simulink library "working_reference_library"  (Simulink 7.9)
settings: Solver=ode45  StartTime=0.0  StopTime=10.0  RelTol=1e-3
undefined symbols (not defined in the file or in its folder): fbaud, fphasej, fsscj, PhaseJ, SSCJ
libraries: simulink_extras x40, working_reference_library x12
Description:
  | Working reference library
settings Model: Creator=asus  LastModifiedBy=asus

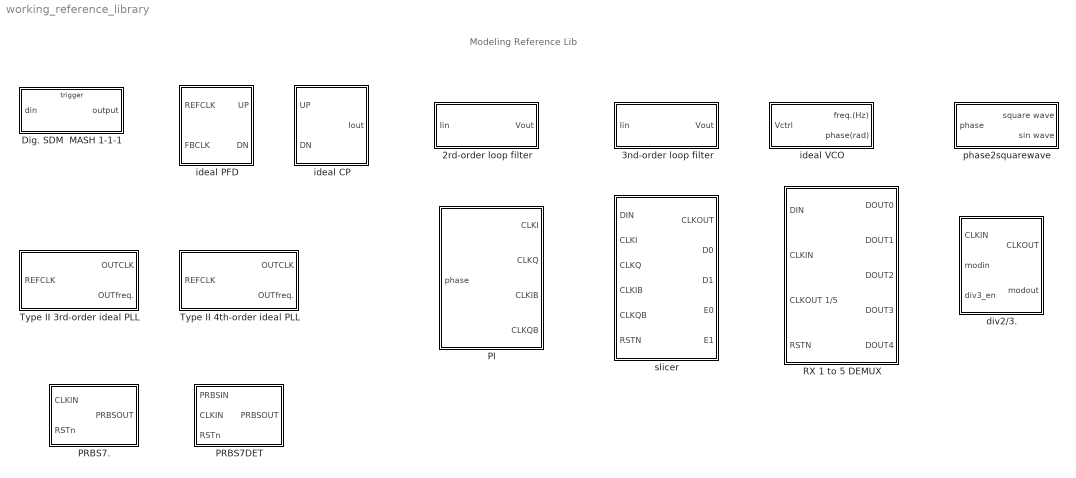
== system working_reference_library ==
  note: Modeling Reference Lib
  2rd-order loop filter : Subsystem  mask{R1=7.5e3, C1=180e-12, C2=4e-12}
      mask prompts: R1 "zero resistor R1(ohm)"; C1 "zero capacitance C1(F)"; C2 "pole capacitance C2(F)"
  3nd-order loop filter : Subsystem  mask{R1=6e3, C1=150e-12, C2=3e-12, R3=6e3*2, C3=1e-12}
      mask prompts: R1 "zero resistor R1(ohm)"; C1 "zero capacitance C1(F)"; C2 "pole1 capacitance C2(F)"; R3 "pole2 resistor R3(ohm)"; C3 "pole2 capacitance C3(F)"
  Dig. SDM  MASH 1-1-1 : Subsystem  TreatAsAtomicUnit=on  mask{N=9}
      mask prompts: N "bit-width for input"
  PI : Subsystem
  PRBS7. : Subsystem
  PRBS7DET : Subsystem
  RX 1 to 5 DEMUX : Subsystem
  Type II 3rd-order ideal PLL : Subsystem  mask{delay=100e-12, Icp=20e-6, R1=6e3, C1=180e-12, C2=4e-12, f_free=1.4e9, Kvco=700e6, Ndiv=15}
      mask prompts: delay "PFD Reset Delay--delay(s)"; Icp "Charge Pump Current--Icp(A)"; R1 "Loop Filter Zero Resistor--R1(ohm)"; C1 "Loop Filter Zero Capacitance--C1(F)"; C2 "Loop Filter Pole Capacitance--C2(F)"; f_free "VCO free running freqency--f_free(Hz)"; Kvco "VCO gain--Kvco(Hz/V)"; Ndiv "Divider Mod--Ndiv"
  Type II 4th-order ideal PLL : Subsystem  mask{delay=100e-12, Icp=20e-6, R1=6e3, C1=180e-12, C2=4e-12, R3=12e3, C3=2e-12, f_free=1.4e9, Kvco=700e6, Ndiv=15}
      mask prompts: delay "PFD Reset Delay--delay(s)"; Icp "Charge Pump Current--Icp(A)"; R1 "Loop Filter Zero resistor--R1(ohm)"; C1 "Loop Filter Zero Capacitance--C1(F)"; C2 "Loop Filter 1st-pole Capacitance--C2(F)"; R3 "Loop Filter 2nd-pole Resistor--R3(ohm)"; C3 "Loop Filter 2nd-pole Capacitance--C3(F)"; f_free "VCO free running freqency--f_free(Hz)"; Kvco "VCO gain--Kvco(Hz/V)"; Ndiv "Divider Mod--Ndiv"
  div2/3. : Subsystem
  ideal CP : Subsystem  mask{Icp=20e-6}
      mask prompts: Icp "charge pump current(A)"
  ideal PFD : Subsystem  mask{delay=100e-12}
      mask prompts: delay "reset delay"
  ideal VCO : Subsystem  mask{f_free=1.4e9, Kvco=700e6}
      mask prompts: f_free "free running freq.(Hz)"; Kvco "VCO gain(Hz/V)"
  phase2squarewave : Subsystem
  slicer : Subsystem  TreatAsAtomicUnit=on

== system working_reference_library/2rd-order loop filter ==
  Iin : Inport
  Data Type Conversion : DataTypeConversion  OutDataTypeStr=double
  Transfer Fcn : TransferFcn  Numerator=[R1*C1 1]  Denominator=[C2*R1*C1 (C1+C2) 0]  AbsoluteTolerance=1e-12
  Vout : Outport
  wires:
  Data Type Conversion/1 -> Transfer Fcn/1
  Transfer Fcn/1 -> Vout/1
  Iin/1 -> Data Type Conversion/1

== system working_reference_library/3nd-order loop filter ==
  Iin : Inport
  Data Type Conversion : DataTypeConversion  OutDataTypeStr=double
  Transfer Fcn : TransferFcn  Numerator=[R1*C1 1]  Denominator=[C2*R1*C1*R3*C3 (C1*R3*C3+C3*R1*C1+C2*(R1*C1+R3*C3)) (C1+C2+C3) 0]  AbsoluteTolerance=1e-12
  Vout : Outport
  wires:
  Iin/1 -> Data Type Conversion/1
  Transfer Fcn/1 -> Vout/1
  Data Type Conversion/1 -> Transfer Fcn/1

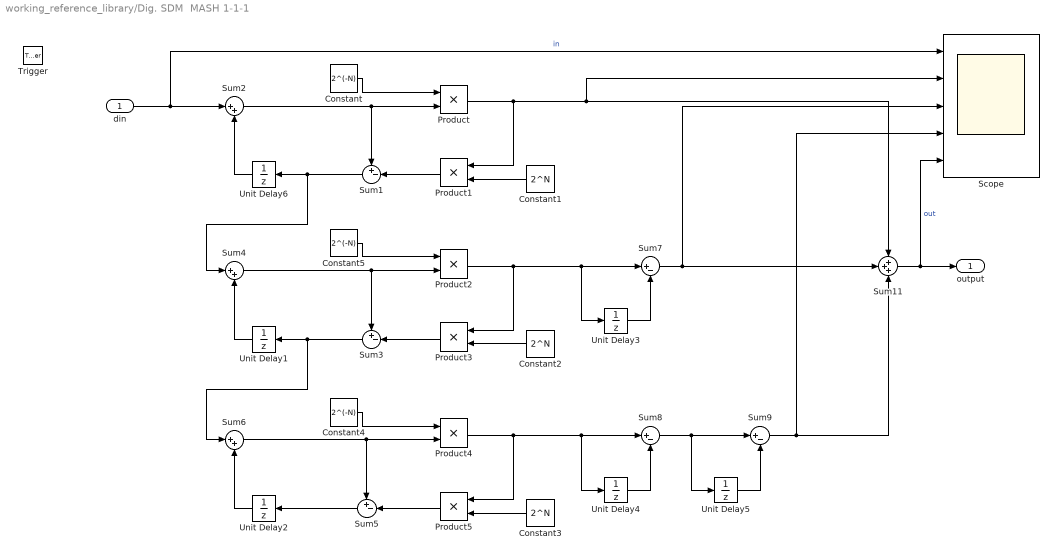
== system working_reference_library/Dig. SDM  MASH 1-1-1 ==
  din : Inport
  Trigger : TriggerPort
  Constant : Constant  Value=2^(-N)
  Constant1 : Constant  Value=2^N
  Constant2 : Constant  Value=2^N
  Constant3 : Constant  Value=2^N
  Constant4 : Constant  Value=2^(-N)
  Constant5 : Constant  Value=2^(-N)
  Product : Product  OutDataTypeStr=int8  RndMeth=Zero
  Product1 : Product  RndMeth=Zero
  Product2 : Product  OutDataTypeStr=int8  RndMeth=Zero
  Product3 : Product  RndMeth=Zero
  Product4 : Product  OutDataTypeStr=int8  RndMeth=Zero
  Product5 : Product  RndMeth=Zero
  Scope : Scope  NumInputPorts=5
      settings: YMin=-100~0~-5~-5~-5  YMax=600~1~5~5~5  MaxDataPoints=500000
  Sum1 : Sum  Inputs=+-|
  Sum11 : Sum  Inputs=+++
  Sum2 : Sum  Inputs=|++
  Sum3 : Sum  Inputs=+-|
  Sum4 : Sum  Inputs=|++
  Sum5 : Sum  Inputs=+-|
  Sum6 : Sum  Inputs=|++
  Sum7 : Sum  Inputs=|+-
  Sum8 : Sum  Inputs=|+-
  Sum9 : Sum  Inputs=|+-
  Unit Delay{1..6} (6 alike) : UnitDelay  SampleTime=-1
  output : Outport
  wires:
  Constant/1 -> Product/1
  Product/1 -> Product1/1, Sum11/1, Scope/2
  Constant1/1 -> Product1/2
  Product1/1 -> Sum1/2
  din/1 -> Sum2/1, Scope/1  "in"
  Sum11/1 -> output/1, Scope/5  "out"
  Unit Delay6/1 -> Sum2/2
  Sum2/1 -> Sum1/1, Product/2
  Constant5/1 -> Product2/1
  Product2/1 -> Product3/1, Sum7/1, Unit Delay3/1
  Constant2/1 -> Product3/2
  Product3/1 -> Sum3/2
  Unit Delay1/1 -> Sum4/2
  Sum4/1 -> Sum3/1, Product2/2
  Constant4/1 -> Product4/1
  Product4/1 -> Product5/1, Sum8/1, Unit Delay4/1
  Constant3/1 -> Product5/2
  Unit Delay2/1 -> Sum6/2
  Sum6/1 -> Sum5/1, Product4/2
  Unit Delay3/1 -> Sum7/2
  Unit Delay4/1 -> Sum8/2
  Sum8/1 -> Sum9/1, Unit Delay5/1
  Unit Delay5/1 -> Sum9/2
  Sum9/1 -> Sum11/3, Scope/4
  Sum7/1 -> Sum11/2, Scope/3
  Sum1/1 -> Unit Delay6/1, Sum4/1
  Product5/1 -> Sum5/2
  Sum5/1 -> Unit Delay2/1
  Sum3/1 -> Unit Delay1/1, Sum6/1

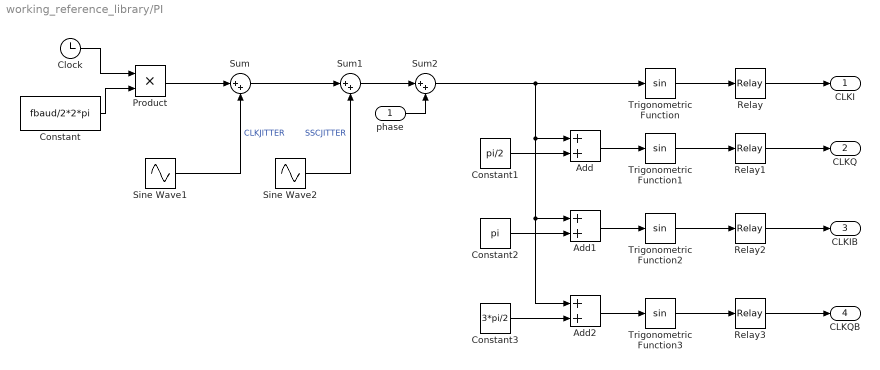
== system working_reference_library/PI ==
  phase : Inport
  Add : Sum
  Add1 : Sum
  Add2 : Sum
  Clock : Clock
  Constant : Constant  Value=fbaud/2*2*pi
  Constant1 : Constant  Value=pi/2
  Constant2 : Constant  Value=pi
  Constant3 : Constant  Value=3*pi/2
  Product : Product  RndMeth=Zero
  Relay{,1..3} (4 alike) : Relay  OnSwitchValue=0.5  OffSwitchValue=-0.5
  Sine Wave1 : Sin  Amplitude=PhaseJ  Frequency=fphasej*2*pi  SampleTime=0
  Sine Wave2 : Sin  Amplitude=SSCJ  Frequency=fsscj*2*pi  SampleTime=0
  Sum : Sum  Inputs=|++
  Sum1 : Sum  Inputs=|++
  Sum2 : Sum  Inputs=|++
  Trigonometric Function{,1..3} (4 alike) : Trigonometry
  CLKI : Outport
  CLKQ : Outport  Port=2
  CLKIB : Outport  Port=3
  CLKQB : Outport  Port=4
  wires:
  Sum2/1 -> Add2/1, Add1/1, Add/1, Trigonometric Function/1
  phase/1 -> Sum2/2
  Sum1/1 -> Sum2/1
  Relay3/1 -> CLKQB/1
  Relay2/1 -> CLKIB/1
  Relay1/1 -> CLKQ/1
  Relay/1 -> CLKI/1
  Add2/1 -> Trigonometric Function3/1
  Trigonometric Function3/1 -> Relay3/1
  Constant3/1 -> Add2/2
  Add1/1 -> Trigonometric Function2/1
  Trigonometric Function2/1 -> Relay2/1
  Constant2/1 -> Add1/2
  Add/1 -> Trigonometric Function1/1
  Trigonometric Function1/1 -> Relay1/1
  Constant1/1 -> Add/2
  Trigonometric Function/1 -> Relay/1
  Sine Wave2/1 -> Sum1/2  "SSCJITTER"
  Sum/1 -> Sum1/1
  Sine Wave1/1 -> Sum/2  "CLKJITTER"
  Product/1 -> Sum/1
  Constant/1 -> Product/2
  Clock/1 -> Product/1

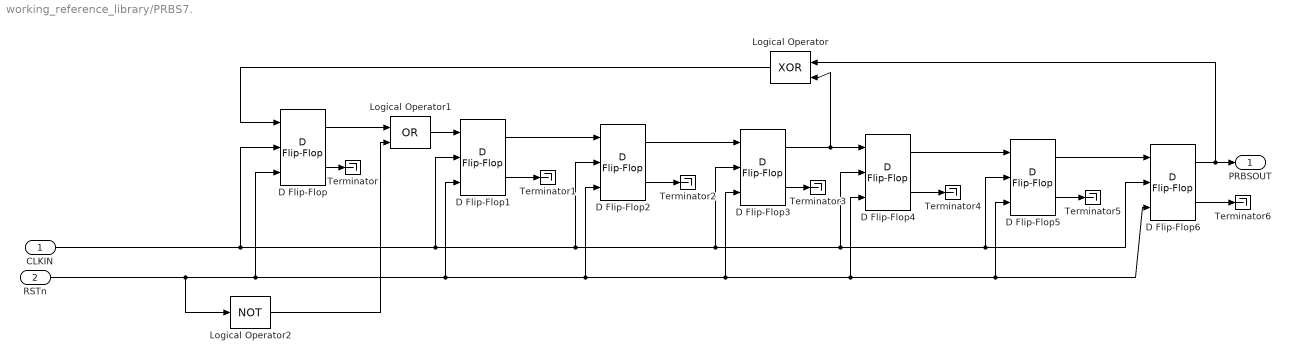
== system working_reference_library/PRBS7. ==
  CLKIN : Inport
  RSTn : Inport  Port=2
  D Flip-Flop{,1..6} (7 alike) : simulink_extras/Flip Flops/D Flip-Flop
  Logical Operator : Logic  Operator=XOR  IconShape=distinctive  AllPortsSameDT=off  OutDataTypeStr=boolean
  Logical Operator1 : Logic  Operator=OR  IconShape=distinctive  AllPortsSameDT=off  OutDataTypeStr=boolean
  Logical Operator2 : Logic  Operator=NOT  IconShape=distinctive  AllPortsSameDT=off  OutDataTypeStr=boolean
  Terminator{,1..6} (7 alike) : Terminator
  PRBSOUT : Outport
  wires:
  Logical Operator2/1 -> Logical Operator1/2
  D Flip-Flop/1 -> Logical Operator1/1
  Logical Operator1/1 -> D Flip-Flop1/1
  D Flip-Flop6/1 -> Logical Operator/1, PRBSOUT/1
  D Flip-Flop6/2 -> Terminator6/1
  D Flip-Flop5/2 -> Terminator5/1
  D Flip-Flop4/2 -> Terminator4/1
  D Flip-Flop3/2 -> Terminator3/1
  D Flip-Flop5/1 -> D Flip-Flop6/1
  D Flip-Flop4/1 -> D Flip-Flop5/1
  D Flip-Flop3/1 -> D Flip-Flop4/1, Logical Operator/2
  RSTn/1 -> D Flip-Flop6/3, D Flip-Flop5/3, D Flip-Flop4/3, D Flip-Flop3/3, D Flip-Flop2/3, D Flip-Flop1/3, D Flip-Flop/3, Logical Operator2/1
  D Flip-Flop2/2 -> Terminator2/1
  D Flip-Flop2/1 -> D Flip-Flop3/1
  D Flip-Flop1/2 -> Terminator1/1
  D Flip-Flop1/1 -> D Flip-Flop2/1
  D Flip-Flop/2 -> Terminator/1
  CLKIN/1 -> D Flip-Flop/2, D Flip-Flop1/2, D Flip-Flop2/2, D Flip-Flop3/2, D Flip-Flop4/2, D Flip-Flop6/2, D Flip-Flop5/2
  Logical Operator/1 -> D Flip-Flop/1

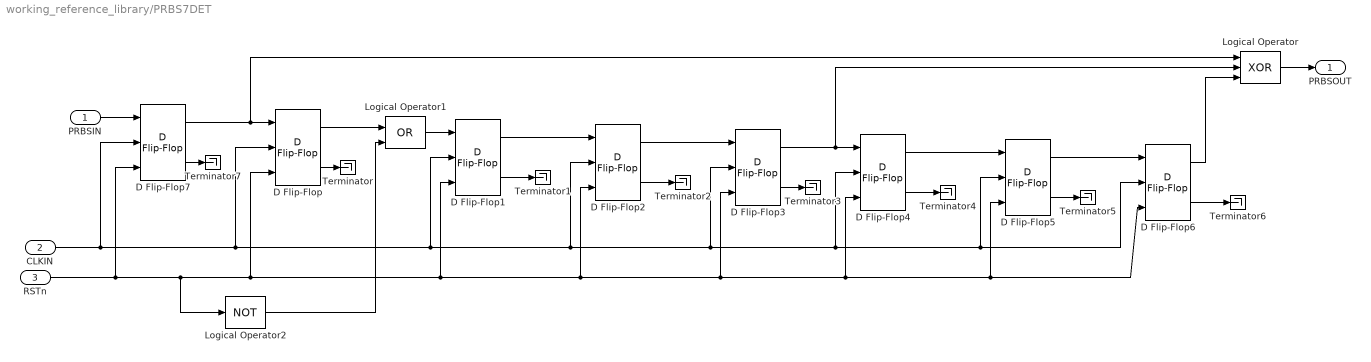
== system working_reference_library/PRBS7DET ==
  PRBSIN : Inport
  CLKIN : Inport  Port=2
  RSTn : Inport  Port=3
  D Flip-Flop{,1..7} (8 alike) : simulink_extras/Flip Flops/D Flip-Flop
  Logical Operator : Logic  Operator=XOR  Inputs=3  IconShape=distinctive  AllPortsSameDT=off  OutDataTypeStr=boolean
  Logical Operator1 : Logic  Operator=OR  IconShape=distinctive  AllPortsSameDT=off  OutDataTypeStr=boolean
  Logical Operator2 : Logic  Operator=NOT  IconShape=distinctive  AllPortsSameDT=off  OutDataTypeStr=boolean
  Terminator{,1..7} (8 alike) : Terminator
  PRBSOUT : Outport
  wires:
  CLKIN/1 -> D Flip-Flop5/2, D Flip-Flop6/2, D Flip-Flop4/2, D Flip-Flop3/2, D Flip-Flop2/2, D Flip-Flop1/2, D Flip-Flop/2, D Flip-Flop7/2
  D Flip-Flop/2 -> Terminator/1
  D Flip-Flop1/1 -> D Flip-Flop2/1
  D Flip-Flop1/2 -> Terminator1/1
  D Flip-Flop2/1 -> D Flip-Flop3/1
  D Flip-Flop2/2 -> Terminator2/1
  RSTn/1 -> Logical Operator2/1, D Flip-Flop/3, D Flip-Flop1/3, D Flip-Flop2/3, D Flip-Flop3/3, D Flip-Flop4/3, D Flip-Flop5/3, D Flip-Flop6/3, D Flip-Flop7/3
  D Flip-Flop3/1 -> D Flip-Flop4/1, Logical Operator/2
  D Flip-Flop4/1 -> D Flip-Flop5/1
  D Flip-Flop5/1 -> D Flip-Flop6/1
  D Flip-Flop3/2 -> Terminator3/1
  D Flip-Flop4/2 -> Terminator4/1
  D Flip-Flop5/2 -> Terminator5/1
  D Flip-Flop6/2 -> Terminator6/1
  D Flip-Flop6/1 -> Logical Operator/3
  Logical Operator1/1 -> D Flip-Flop1/1
  D Flip-Flop/1 -> Logical Operator1/1
  Logical Operator2/1 -> Logical Operator1/2
  D Flip-Flop7/1 -> D Flip-Flop/1, Logical Operator/1
  D Flip-Flop7/2 -> Terminator7/1
  Logical Operator/1 -> PRBSOUT/1
  PRBSIN/1 -> D Flip-Flop7/1

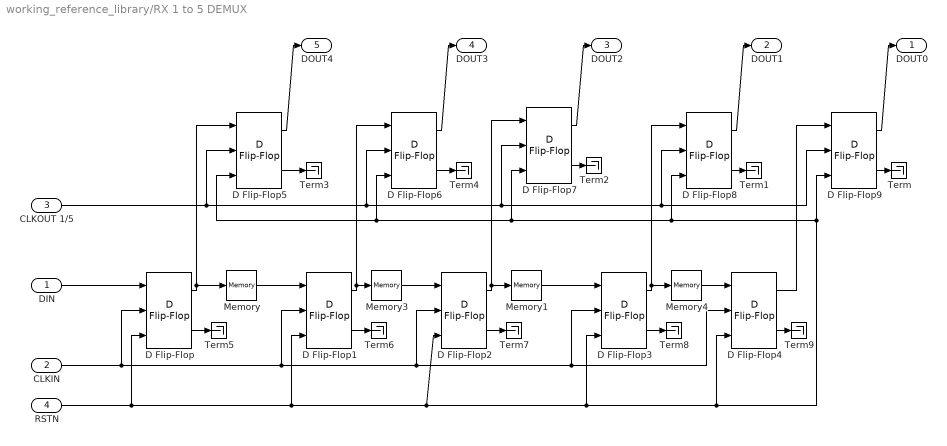
== system working_reference_library/RX 1 to 5 DEMUX ==
  DIN : Inport
  CLKIN : Inport  Port=2
  CLKOUT 1/5 : Inport  Port=3
  RSTN : Inport  Port=4
  D Flip-Flop{,1..9} (10 alike) : simulink_extras/Flip Flops/D Flip-Flop
  Memory{,1,3..4} (4 alike) : Memory
  Term{,1..9} (10 alike) : Terminator
  DOUT0 : Outport
  DOUT1 : Outport  Port=2
  DOUT2 : Outport  Port=3
  DOUT3 : Outport  Port=4
  DOUT4 : Outport  Port=5
  wires:
  DIN/1 -> D Flip-Flop/1
  D Flip-Flop/1 -> Memory/1, D Flip-Flop5/1
  Memory/1 -> D Flip-Flop1/1
  D Flip-Flop1/1 -> D Flip-Flop6/1, Memory3/1
  D Flip-Flop2/1 -> D Flip-Flop7/1, Memory1/1
  Memory1/1 -> D Flip-Flop3/1
  D Flip-Flop3/1 -> D Flip-Flop8/1, Memory4/1
  Memory3/1 -> D Flip-Flop2/1
  Memory4/1 -> D Flip-Flop4/1
  D Flip-Flop5/1 -> DOUT4/1
  D Flip-Flop4/1 -> D Flip-Flop9/1
  D Flip-Flop6/1 -> DOUT3/1
  D Flip-Flop7/1 -> DOUT2/1
  D Flip-Flop8/1 -> DOUT1/1
  D Flip-Flop9/1 -> DOUT0/1
  CLKOUT 1/5/1 -> D Flip-Flop9/2, D Flip-Flop8/2, D Flip-Flop7/2, D Flip-Flop6/2, D Flip-Flop5/2
  CLKIN/1 -> D Flip-Flop4/2, D Flip-Flop3/2, D Flip-Flop2/2, D Flip-Flop1/2, D Flip-Flop/2
  RSTN/1 -> D Flip-Flop/3, D Flip-Flop1/3, D Flip-Flop2/3, D Flip-Flop3/3, D Flip-Flop4/3, D Flip-Flop9/3, D Flip-Flop8/3, D Flip-Flop7/3, D Flip-Flop5/3, D Flip-Flop6/3
  D Flip-Flop9/2 -> Term/1
  D Flip-Flop7/2 -> Term2/1
  D Flip-Flop5/2 -> Term3/1
  D Flip-Flop6/2 -> Term4/1
  D Flip-Flop8/2 -> Term1/1
  D Flip-Flop4/2 -> Term9/1
  D Flip-Flop3/2 -> Term8/1
  D Flip-Flop2/2 -> Term7/1
  D Flip-Flop1/2 -> Term6/1
  D Flip-Flop/2 -> Term5/1

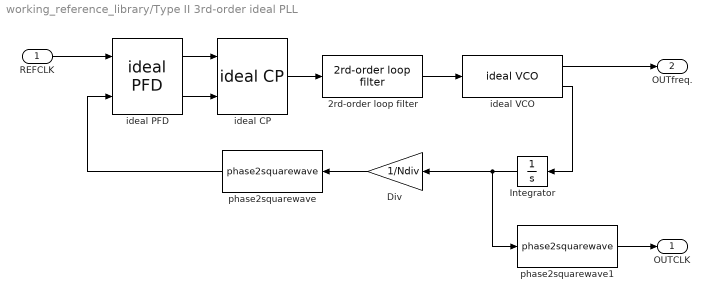
== system working_reference_library/Type II 3rd-order ideal PLL ==
  REFCLK : Inport
  2rd-order loop filter : working_reference_library/2rd-order loop filter  R1=R1  C1=C1  C2=C2
  Div : Gain  Gain=1/Ndiv
  Integrator : Integrator
  ideal CP : working_reference_library/ideal CP  Icp=Icp
  ideal PFD : working_reference_library/ideal PFD  delay=delay
  ideal VCO : working_reference_library/ideal VCO  f_free=f_free  Kvco=Kvco
  phase2squarewave : working_reference_library/phase2squarewave
  phase2squarewave1 : working_reference_library/phase2squarewave
  OUTCLK : Outport
  OUTfreq. : Outport  Port=2
  wires:
  ideal PFD/1 -> ideal CP/1
  ideal PFD/2 -> ideal CP/2
  ideal CP/1 -> 2rd-order loop filter/1
  2rd-order loop filter/1 -> ideal VCO/1
  REFCLK/1 -> ideal PFD/1
  phase2squarewave/1 -> ideal PFD/2
  ideal VCO/2 -> Integrator/1
  Integrator/1 -> Div/1, phase2squarewave1/1
  Div/1 -> phase2squarewave/1
  phase2squarewave1/1 -> OUTCLK/1
  ideal VCO/1 -> OUTfreq./1

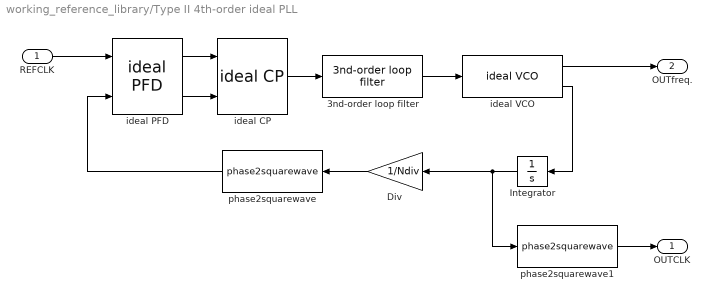
== system working_reference_library/Type II 4th-order ideal PLL ==
  REFCLK : Inport
  3nd-order loop filter : working_reference_library/3nd-order loop filter  R1=R1  C1=C1  C2=C2  R3=R3  C3=C3
  Div : Gain  Gain=1/Ndiv
  Integrator : Integrator
  ideal CP : working_reference_library/ideal CP  Icp=Icp
  ideal PFD : working_reference_library/ideal PFD  delay=delay
  ideal VCO : working_reference_library/ideal VCO  f_free=f_free  Kvco=Kvco
  phase2squarewave : working_reference_library/phase2squarewave
  phase2squarewave1 : working_reference_library/phase2squarewave
  OUTCLK : Outport
  OUTfreq. : Outport  Port=2
  wires:
  ideal PFD/1 -> ideal CP/1
  ideal PFD/2 -> ideal CP/2
  ideal CP/1 -> 3nd-order loop filter/1
  3nd-order loop filter/1 -> ideal VCO/1
  REFCLK/1 -> ideal PFD/1
  phase2squarewave/1 -> ideal PFD/2
  ideal VCO/2 -> Integrator/1
  Integrator/1 -> Div/1, phase2squarewave1/1
  Div/1 -> phase2squarewave/1
  phase2squarewave1/1 -> OUTCLK/1
  ideal VCO/1 -> OUTfreq./1

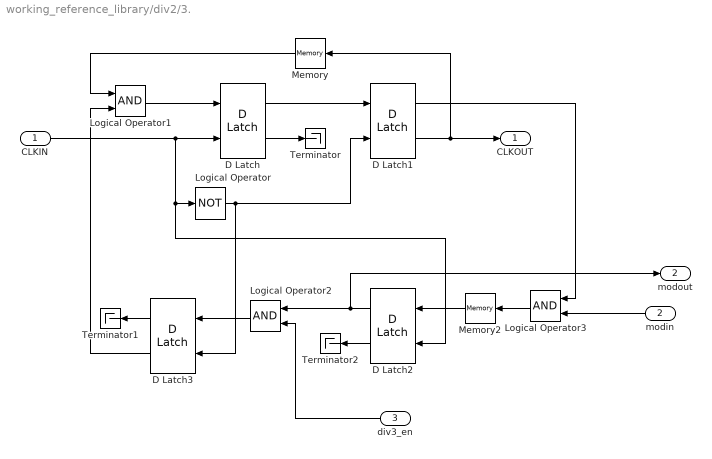
== system working_reference_library/div2/3. ==
  CLKIN : Inport
  modin : Inport  Port=2
  div3_en : Inport  Port=3
  D Latch{,1..3} (4 alike) : simulink_extras/Flip Flops/D Latch
  Logical Operator : Logic  Operator=NOT  AllPortsSameDT=off  OutDataTypeStr=boolean
  Logical Operator1 : Logic  AllPortsSameDT=off  OutDataTypeStr=boolean
  Logical Operator2 : Logic  AllPortsSameDT=off  OutDataTypeStr=boolean
  Logical Operator3 : Logic  AllPortsSameDT=off  OutDataTypeStr=boolean
  Memory : Memory
  Memory2 : Memory
  Terminator : Terminator
  Terminator1 : Terminator
  Terminator2 : Terminator
  CLKOUT : Outport
  modout : Outport  Port=2
  wires:
  D Latch/1 -> D Latch1/1
  Logical Operator/1 -> D Latch1/2, D Latch3/2
  D Latch1/2 -> CLKOUT/1, Memory/1
  Logical Operator1/1 -> D Latch/1
  Memory/1 -> Logical Operator1/1
  D Latch2/1 -> Logical Operator2/1, modout/1
  D Latch1/1 -> Logical Operator3/1
  Logical Operator3/1 -> Memory2/1
  div3_en/1 -> Logical Operator2/2
  Logical Operator2/1 -> D Latch3/1
  CLKIN/1 -> D Latch/2, Logical Operator/1, D Latch2/2
  D Latch3/2 -> Logical Operator1/2
  Memory2/1 -> D Latch2/1
  modin/1 -> Logical Operator3/2
  D Latch/2 -> Terminator/1
  D Latch3/1 -> Terminator1/1
  D Latch2/2 -> Terminator2/1

== system working_reference_library/ideal CP ==
  UP : Inport
  DN : Inport  Port=2
  Add : Sum  Inputs=+-
  Icp : Gain  Gain=Icp
  Iout : Outport
  wires:
  UP/1 -> Add/1
  DN/1 -> Add/2
  Add/1 -> Icp/1
  Icp/1 -> Iout/1

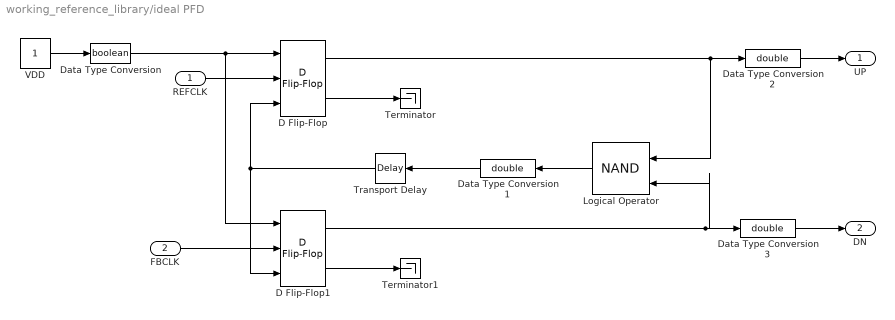
== system working_reference_library/ideal PFD ==
  REFCLK : Inport
  FBCLK : Inport  Port=2
  D Flip-Flop : simulink_extras/Flip Flops/D Flip-Flop
  D Flip-Flop1 : simulink_extras/Flip Flops/D Flip-Flop
  Data Type Conversion : DataTypeConversion  OutDataTypeStr=boolean
  Data Type Conversion1 : DataTypeConversion  OutDataTypeStr=double
  Data Type Conversion2 : DataTypeConversion  OutDataTypeStr=double
  Data Type Conversion3 : DataTypeConversion  OutDataTypeStr=double
  Logical Operator : Logic  Operator=NAND  IconShape=distinctive  AllPortsSameDT=off  OutDataTypeStr=boolean
  Terminator : Terminator
  Terminator1 : Terminator
  Transport Delay : TransportDelay  DelayTime=delay
  VDD : Constant
  UP : Outport
  DN : Outport  Port=2
  wires:
  REFCLK/1 -> D Flip-Flop/2
  FBCLK/1 -> D Flip-Flop1/2
  D Flip-Flop/1 -> Logical Operator/1, Data Type Conversion2/1
  D Flip-Flop1/1 -> Logical Operator/2, Data Type Conversion3/1
  Logical Operator/1 -> Data Type Conversion1/1
  Transport Delay/1 -> D Flip-Flop1/3, D Flip-Flop/3
  VDD/1 -> Data Type Conversion/1
  Data Type Conversion/1 -> D Flip-Flop/1, D Flip-Flop1/1
  Data Type Conversion1/1 -> Transport Delay/1
  Data Type Conversion2/1 -> UP/1
  Data Type Conversion3/1 -> DN/1
  D Flip-Flop/2 -> Terminator/1
  D Flip-Flop1/2 -> Terminator1/1

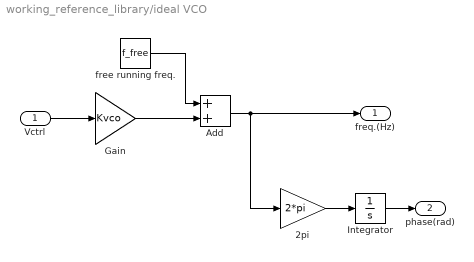
== system working_reference_library/ideal VCO ==
  Vctrl : Inport
  2pi : Gain  Gain=2*pi
  Add : Sum
  Gain : Gain  Gain=Kvco
  Integrator : Integrator
  free running freq. : Constant  Value=f_free
  freq.(Hz) : Outport
  phase(rad) : Outport  Port=2
  wires:
  free running freq./1 -> Add/1
  Vctrl/1 -> Gain/1
  Gain/1 -> Add/2
  Add/1 -> freq.(Hz)/1, 2pi/1
  2pi/1 -> Integrator/1
  Integrator/1 -> phase(rad)/1

== system working_reference_library/phase2squarewave ==
  phase : Inport
  Relay : Relay  OnSwitchValue=0.5  OffSwitchValue=-0.5
  Trigonometric Function : Trigonometry
  square wave : Outport
  sin wave : Outport  Port=2
  wires:
  Trigonometric Function/1 -> Relay/1, sin wave/1
  phase/1 -> Trigonometric Function/1
  Relay/1 -> square wave/1

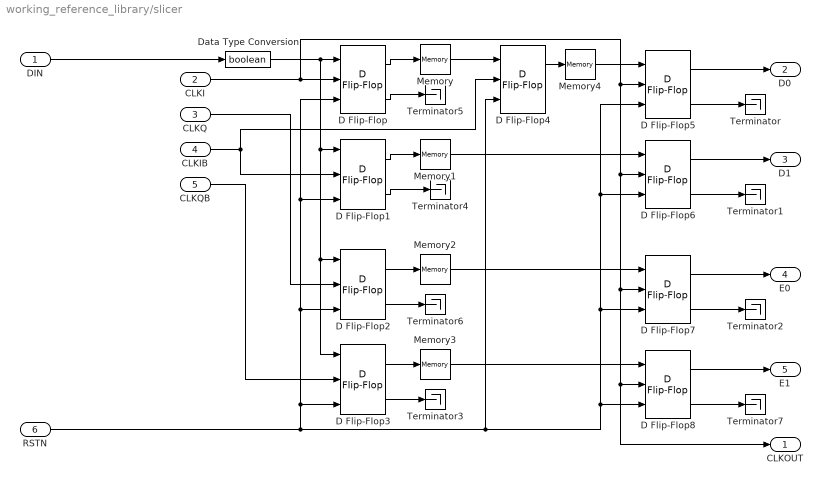
== system working_reference_library/slicer ==
  DIN : Inport
  CLKI : Inport  Port=2
  CLKQ : Inport  Port=3
  CLKIB : Inport  Port=4
  CLKQB : Inport  Port=5
  RSTN : Inport  Port=6
  D Flip-Flop{,1..8} (9 alike) : simulink_extras/Flip Flops/D Flip-Flop
  Data Type Conversion : DataTypeConversion  OutDataTypeStr=boolean
  Memory{,1..4} (5 alike) : Memory
  Terminator{,1..7} (8 alike) : Terminator
  CLKOUT : Outport
  D0 : Outport  Port=2
  D1 : Outport  Port=3
  E0 : Outport  Port=4
  E1 : Outport  Port=5
  wires:
  Memory4/1 -> D Flip-Flop5/1
  D Flip-Flop8/1 -> E1/1
  Memory3/1 -> D Flip-Flop8/1
  D Flip-Flop4/1 -> Memory4/1
  Memory1/1 -> D Flip-Flop6/1
  Memory2/1 -> D Flip-Flop7/1
  RSTN/1 -> D Flip-Flop4/3, D Flip-Flop6/3, D Flip-Flop5/3, D Flip-Flop7/3, D Flip-Flop8/3, D Flip-Flop3/3, D Flip-Flop2/3, D Flip-Flop1/3, D Flip-Flop/3
  D Flip-Flop2/2 -> Terminator6/1
  D Flip-Flop/2 -> Terminator5/1
  D Flip-Flop1/2 -> Terminator4/1
  D Flip-Flop3/2 -> Terminator3/1
  D Flip-Flop7/2 -> Terminator2/1
  D Flip-Flop6/2 -> Terminator1/1
  D Flip-Flop5/2 -> Terminator/1
  Memory/1 -> D Flip-Flop4/1
  Data Type Conversion/1 -> D Flip-Flop/1, D Flip-Flop1/1, D Flip-Flop3/1, D Flip-Flop2/1
  D Flip-Flop3/1 -> Memory3/1
  D Flip-Flop7/1 -> E0/1
  D Flip-Flop2/1 -> Memory2/1
  CLKQ/1 -> D Flip-Flop2/2
  D Flip-Flop6/1 -> D1/1
  D Flip-Flop5/1 -> D0/1
  DIN/1 -> Data Type Conversion/1
  CLKQB/1 -> D Flip-Flop3/2
  D Flip-Flop1/1 -> Memory1/1
  D Flip-Flop/1 -> Memory/1
  CLKIB/1 -> D Flip-Flop4/2, D Flip-Flop1/2
  CLKI/1 -> D Flip-Flop7/2, D Flip-Flop8/2, CLKOUT/1, D Flip-Flop6/2, D Flip-Flop5/2, D Flip-Flop/2
  D Flip-Flop8/2 -> Terminator7/1
